simulink model "PID_SpringDamper"  (R2021a)
settings: Solver=VariableStepAuto  StartTime=0.0  StopTime=sim_time  MaxStep=step_value  RelTol=1e-3
values from neighbouring files (symbols this model uses):
  b = 3.5077E-6    (= 3.5077e-06)    [DCMotor_reduction_run.m]    (also in DCMotor_run.m; MassSpringDamper_run.m = 2; PID_ScriptOnly.m = 50; PID_SpringDamper_run.m = 10)
  F = 1    [MassSpringDamper_run.m]    (also in PID_SpringDamper_run.m = 10; TrainSimulation_run.m; TransferFunctionModel_run.m = 10)
  k = 20    [MassSpringDamper_run.m]    (also in PID_SpringDamper_run.m; PID_block_run.m; TrainSimulation_run.m = 1; TransferFunctionModel_run.m)
  Kd = 0    [DCMotor_reduction_run.m]    (also in PID_SpringDamper_run.m = 50; PID_block_run.m; PID_vehicle_run.m)
  Ki = 1    [DCMotor_reduction_run.m]    (also in PID_ScriptOnly.m = 40; PID_SpringDamper_run.m = 300; PID_block_run.m = 0; PID_vehicle_run.m)
  Kp = 0.5    [DCMotor_reduction_run.m]    (also in PID_ScriptOnly.m = 800; PID_SpringDamper_run.m = 350; PID_block_run.m = 1000; PID_vehicle_run.m = 1)
  M = 1    [MassSpringDamper_run.m]    (also in PID_SpringDamper_run.m; PID_block_run.m; PID_vehicle_run.m; TransferFunctionModel_run.m)
settings Model: Creator=shinyh  LastModifiedBy=shinyh

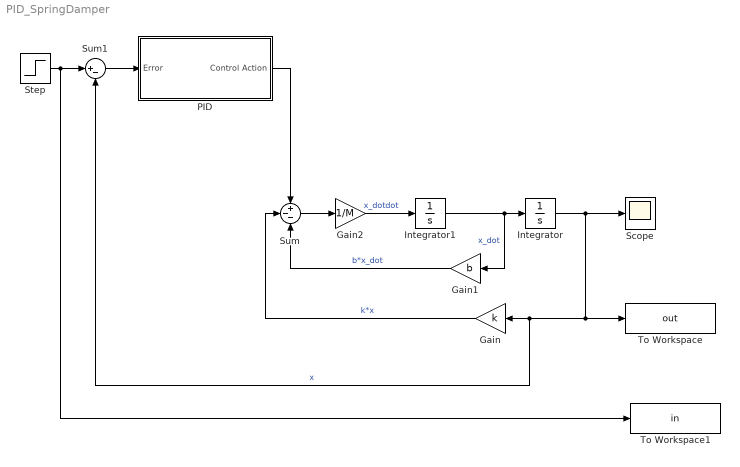
== system PID_SpringDamper ==
  Gain : Gain  Gain=k
  Gain1 : Gain  Gain=b
  Gain2 : Gain  Gain=1/M
  Integrator : Integrator
  Integrator1 : Integrator
  PID : Subsystem
  Scope : Scope
  Step : Step  After=F  SampleTime=0
  Sum : Sum  Inputs=+--
  Sum1 : Sum  Inputs=|+-
  To Workspace : ToWorkspace  VariableName=out  SaveFormat=Timeseries  SampleTime=-1
  To Workspace1 : ToWorkspace  VariableName=in  SaveFormat=Timeseries  SampleTime=-1
  wires:
  Gain/1 -> Sum/2  "k*x"
  Integrator1/1 -> Gain1/1, Integrator/1  "x_dot"
  Sum/1 -> Gain2/1
  Gain2/1 -> Integrator1/1  "x_dotdot"
  PID/1(Control Action) -> Sum/1
  Gain1/1 -> Sum/3  "b*x_dot"
  Integrator/1 -> To Workspace/1, Sum1/2, Gain/1, Scope/1  "x"
  Step/1 -> To Workspace1/1, Sum1/1
  Sum1/1 -> PID/1(Error)

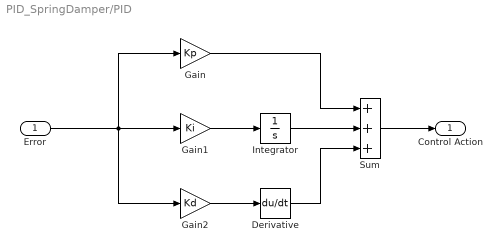
== system PID_SpringDamper/PID ==
  Error : Inport
  Derivative : Derivative
  Gain : Gain  Gain=Kp
  Gain1 : Gain  Gain=Ki
  Gain2 : Gain  Gain=Kd
  Integrator : Integrator
  Sum : Sum  Inputs=+++
  Control Action : Outport
  wires:
  Sum/1 -> Control Action/1
  Gain2/1 -> Derivative/1
  Integrator/1 -> Sum/2
  Gain1/1 -> Integrator/1
  Gain/1 -> Sum/1
  Error/1 -> Gain2/1, Gain1/1, Gain/1
  Derivative/1 -> Sum/3
